simulink model "Golf_Lin_MIMO"  (R2019a)
settings: Solver=VariableStepAuto  StartTime=0.0  StopTime=300  RelTol=1e-3
values from neighbouring files (symbols this model uses):
  DEG2RAD = pi/180.    (= 0.0174532925199)    [mainProjetCADV_2a.m]    (also in utAcDynamicsFunction.m; utConstantAeroCoeff.m)
  KTS2MS = 1852 / 3600    (= 0.514444444444)    [mainProjetCADV_2a.m]    (also in utAcDynamicsFunction.m)
undefined symbols (not defined in the file or in its folder): A_sys, Ar, B_sys, Br, C_sys, Cr, D_sys, Dpf, Dr, Kr, Kx
settings Model: Creator=ulyss  LastModifiedBy=ulyss

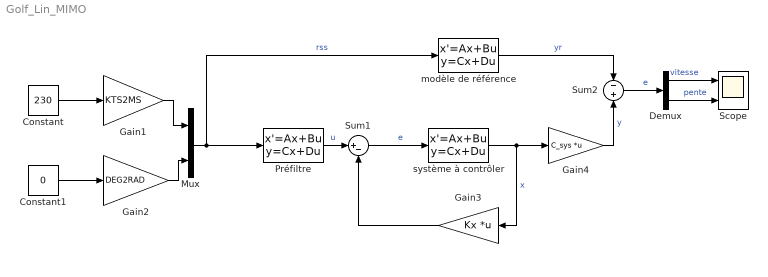
== system Golf_Lin_MIMO ==
  Constant : Constant  Value=230
  Constant1 : Constant  Value=0
  Demux : Demux  Outputs=2
  Gain1 : Gain  Gain=KTS2MS
  Gain2 : Gain  Gain=DEG2RAD
  Gain3 : Gain  Gain=Kx  Multiplication=Matrix(K*u) (u vector)
  Gain4 : Gain  Gain=C_sys  Multiplication=Matrix(K*u) (u vector)
  Mux : Mux  Inputs=2
  Préfiltre : StateSpace  A=Ar  B=Br  C=-Kr  D=Dpf  InitialCondition=0
  Scope : Scope  NumInputPorts=2
  Sum1 : Sum  Inputs=|+-
  Sum2 : Sum  Inputs=-|+
  modèle de référence : StateSpace  A=Ar  B=Br  C=Cr  D=Dr  InitialCondition=0
  système à contrôler : StateSpace  A=A_sys  B=B_sys  C=eye(4)  D=D_sys  InitialCondition=0
  wires:
  Constant/1 -> Gain1/1
  Gain1/1 -> Mux/1
  Constant1/1 -> Gain2/1
  Gain2/1 -> Mux/2
  Mux/1 -> Préfiltre/1, modèle de référence/1  "rss"
  Préfiltre/1 -> Sum1/1  "u"
  système à contrôler/1 -> Gain4/1, Gain3/1  "x"
  modèle de référence/1 -> Sum2/1  "yr"
  Sum2/1 -> Demux/1  "e"
  Gain4/1 -> Sum2/2  "y"
  Gain3/1 -> Sum1/2
  Sum1/1 -> système à contrôler/1  "e"
  Demux/1 -> Scope/1  "vitesse"
  Demux/2 -> Scope/2  "pente"
